simulink model "BMS_MIL_Wrapper"  (R2025b)
settings: Solver=ode3  StartTime=0.0  StopTime=20  FixedStep=.001  RelTol=1e-3  EnableMultiTasking=on
InitFcn:
  | battery_init;
  | Full_Charge_Volt=4.2; % unit volts
  | Cutoff_Volt=3; % unit volts
  | Delta=.02;
  | ContactorTime=20;
  | ContactorTimeOut=100;
  | High_TempLim=333;
  | Low_TempLim=263;
  | Sensor_Fault_Treshold=.02;
  | CurrentTimeout=1;
  | Allowed_Delta=.04;
  | Bal_On_Time=30;
  | Bal_Off_Time=5;
  | BalNotAct_Time=10;
values from neighbouring files (symbols this model uses):
  bonka_R0 = [ ... (first row only)    [battery_init.m]
  bonka_SOC = [0, 0.1, 0.2, 0.3, 0.4, 0.5, 0.6, 0.7, 0.8, 0.9, 1.0]    [battery_init.m]
  bonka_T = [263.15, 273.15, 298.15, 313.15, 328.15]    [battery_init.m]
  Charge_Rate = 1    [battery_init.m]
  Discharge_Rate = -1    [battery_init.m]
  Fly_Cycle_Current = [ ... (first row only)    [battery_init.m]
undefined symbols (not defined in the file or in its folder): DiscIntNeverNeededParam, From_Plant_MATLABStruct, SRE
libraries: fl_lib x69, nesl_utility x54, simulink x35, ee_lib x12, batteryecm_lib x12, BatteryCurrentManagement x1
(part 4 of 4)

== stateflow chart BMS_MIL_Wrapper/Test Sequence ==
  state Charging
    State_Required=SRE.Charge
  (default) -> Charging
  data: State_Required output Enum: SRE

== stateflow chart BMS_MIL_Wrapper/BMS_Closedloop/BMS_Control/Fault_Severity/Chart ==
  state UV_Fault_Severity
    during:
    if UV_Critical
    Fault_Level.UV = 4;
    elseif UV_Emergency
    Fault_Level.UV = 3;
    elseif UV_PowerLimit
    Fault_Level.UV = 2;
    elseif UV_Warning
    Fault_Level.UV = 1;
    else
    Fault_Level.UV = 0;
    end
  (default) -> UV_Fault_Severity
  data: UV_Warning input boolean; UV_PowerLimit input boolean; UV_Emergency input boolean; UV_Critical input boolean; Fault_Level output Bus: Fault_Level

== stateflow chart BMS_MIL_Wrapper/BMS_Closedloop/BMS_Control/Fault_Severity/Chart1 ==
  state UV_Fault_Severity
    during:
    if OV_Critical
    Fault_Level.OV = 3;
    elseif OV_Stop_Charge
    Fault_Level.OV = 2;
    elseif OV_Warning
    Fault_Level.OV= 1;
    else
    Fault_Level.OV = 0;
    end
  (default) -> UV_Fault_Severity
  data: OV_Warning input boolean; OV_Stop_Charge input boolean; OV_Critical input boolean; Fault_Level output Bus: Fault_Level

== stateflow chart BMS_MIL_Wrapper/BMS_Closedloop/BMS_Control/Fault_Severity/Chart2 ==
  state UV_Fault_Severity
    during:
    if OT_Critical
    Fault_Level.OT = 4;
    elseif OT_Emergency
    Fault_Level.OT = 3;
    elseif OT_PowerLimit
    Fault_Level.OT = 2;
    elseif OT_Warning
    Fault_Level.OT = 1;
    else
    Fault_Level.OT = 0;
    end
  (default) -> UV_Fault_Severity
  data: OT_Warning input boolean; OT_PowerLimit input boolean; OT_Emergency input boolean; OT_Critical input boolean; Fault_Level output Bus: Fault_Level

== stateflow chart BMS_MIL_Wrapper/BMS_Closedloop/BMS_Control/Fault_Severity/Chart3 ==
  state UV_Fault_Severity
    during:
    if UT_Critical
    Fault_Level.UT = 4;
    elseif UT_Emergency
    Fault_Level.UT = 3;
    elseif UT_PowerLimit
    Fault_Level.UT = 2;
    elseif UT_Warning
    Fault_Level.UT = 1;
    else
    Fault_Level.UT = 0;
    end
  (default) -> UV_Fault_Severity
  data: UT_Warning input boolean; UT_PowerLimit input boolean; UT_Emergency input boolean; UT_Critical input boolean; Fault_Level output Bus: Fault_Level

== stateflow chart BMS_MIL_Wrapper/BMS_Closedloop/BMS_Control/Subsystem/BMS_States ==
  state Fault_Monitoring [parallel]
    settings: executionOrder=2
    state Monitor_CurrentLim [parallel]
      settings: executionOrder=1
      state No_CurrentLim_Fault
      state Wait
      state OC_Fault
        en:
        FaultPresent=true;
        Fault_out.OC=true;
      (default) -> No_CurrentLim_Fault : {FaultPresent=false;
          |  Fault_out.OC=false;}
      No_CurrentLim_Fault -> Wait : [(Pack_Current< Current_Limits.Discharge_Current_Limit) || ...
          | (Pack_Current> Current_Limits.Charge_Current_Limit)]
      Wait -> No_CurrentLim_Fault [order 2] : [(Pack_Current >= Current_Limits.Discharge_Current_Limit) && ...
          | (Pack_Current <= Current_Limits.Charge_Current_Limit)]
      Wait -> OC_Fault [order 1] : [after(CurrentTimeout, sec)]
    state Monitor_CellVolt [parallel]
      settings: executionOrder=2
      state No_OV_UV
        en,du:
        Delta=abs(V_Batt_Sum-V_Batt_Monitor);
      state OV_Fault
        en:
        FaultPresent=true;
        Fault_out.OV=true;
      state UV_Fault
        en:
        FaultPresent=true;
        Fault_out.UV=true;
      state Sensor_Fault
        en:
        FaultPresent=true;
        Fault_out.VoltSensor=true;
      (default) -> No_OV_UV : {FaultPresent=false;
          | Fault_out.VoltSensor=false;
          | Fault_out.UV=false;
          | Fault_out.OV=false;}
      No_OV_UV -> OV_Fault [order 3] : [Max_Voltage>=Full_Charge_Volt]
      No_OV_UV -> (junction 190) [order 2] : [Min_Voltage <= Cutoff_Volt]
      (junction 190) -> UV_Fault
      No_OV_UV -> Sensor_Fault [order 1] : [Delta>=single(Sensor_Fault_Treshold)]
    state Monitor_CellTemp [parallel]
      settings: executionOrder=3
      state OT_Fault
        en:
        FaultPresent=true;
        Fault_out.OT=true;
      state No_OT_UT
        en, du:
        MaxCellTemp=max(Tmod);
        MinCellTemp=min(Tmod);
      state UT_Fault
        en:
        FaultPresent=true;
        Fault_out.UT=true;
      No_OT_UT -> OT_Fault [order 2] : [MaxCellTemp>=High_TempLim]
      (default) -> No_OT_UT : {FaultPresent=false;
          | Fault_out.OT=false;
          | Fault_out.UT=false;}
      No_OT_UT -> UT_Fault [order 1] : [MinCellTemp<=Low_TempLim]
  state Normal_State [parallel]
    settings: executionOrder=1
    state Standby
      en:
      BMS_State_Out= BMS_State.Standbying
    state Charging
      en:
      BMS_State_Out= BMS_State.Charging
    state Flying
      en:
      BMS_State_Out= BMS_State.Flying
    state Fault
      en,du:
      BMS_State_Out= BMS_State.Fault
    (default) -> Standby
    Standby -> Charging [order 2] : [State_Required==SRE.Charge ]
    Standby -> (junction 206) [order 3] : [FaultPresent]
    (junction 206) -> (junction 209)
    Charging -> Standby [order 1] : [(State_Required~=SRE.Charge)...
        | || (State_Required==SRE.Standby) ]
    Standby -> Flying [order 1] : [State_Required== SRE.Fly]
    Flying -> Standby [order 1] : [(State_Required~=SRE.Fly) ||...
        | (State_Required==SRE.Standby) ]
    (junction 207) -> Charging
    Charging -> (junction 208) [order 2]
    Charging -> Fault [order 3] : [FaultPresent]
    Flying -> (junction 207) [order 2] : [State_Required==SRE.Charge]
    (junction 208) -> Flying : [State_Required== SRE.Fly]
    Flying -> Fault [order 3] : [FaultPresent]
    (junction 209) -> Fault
  data: Current_Limits input Bus: Current_Limits; Tmod input single; V_Batt_Sum input; Pack_Current input single; V_Batt_Monitor input; State_Required input Enum: SRE; Fault_out output Bus: Fault_out; Max_Voltage input single; Min_Voltage input single; Low_TempLim parameter single; High_TempLim parameter single; Cutoff_Volt parameter single; Full_Charge_Volt parameter single; MaxCellTemp local single; MinCellTemp local single; Delta local single; Sensor_Fault_Treshold parameter double; FaultPresent local boolean; BMS_State_Out output Enum: BMS_State; CurrentTimeout parameter

== stateflow chart BMS_MIL_Wrapper/BMS_Closedloop/BMS_Control/Subsystem1/Chart ==
  state Balancing_Off
    en:
    Bal_Cmd(:,:)= false;
    en, du:
    DeltaCellVolt=Max_Voltage-Min_Voltage;
  state Balancing_On
    en, du:
    DeltaCellVolt=Max_Voltage-Min_Voltage;
    state Balance_Active
      en, du:
      Bal_Cmd=((Vmod-Min_Voltage)> Allowed_Delta/2)';
      flgBalCompl=all(~Bal_Cmd);
    state Balance_Not_Active
    (default) -> Balance_Active
    Balance_Not_Active -> Balance_Active [order 1] : [after(BalNotAct_Time, sec) &&...
        |  DeltaCellVolt> Allowed_Delta]
    Balance_Active -> Balance_Not_Active : [flgBalCompl]
  (default) -> Balancing_Off : {flgBalCompl=true}
  Balancing_Off -> Balancing_On : [flgBalInt &&...
      | BMS_State_Out==BMS_State.Charging &&...
      | after(Bal_Off_Time, sec) &&...
      | DeltaCellVolt> Allowed_Delta]
  Balancing_On -> Balancing_Off : [BMS_State_Out==BMS_State.Flying]
  Balance_Not_Active -> Balancing_Off [order 2] : [after(Bal_On_Time, sec)]
  data: BMS_State_Out input; Min_Voltage input single; Max_Voltage input single; Bal_Cmd output boolean; Allowed_Delta parameter single; DeltaCellVolt local single; Bal_On_Time parameter single; Bal_Off_Time parameter single; BalNotAct_Time parameter single; Vmod input single; flgBalCompl local boolean =false; flgBalInt local =true

== stateflow chart BMS_MIL_Wrapper/BMS_Closedloop/FC/Chart ==
  state Needed_Action
    if Fault_Level == 4
    Drone_Mode = 4;
    Motor_Command = 0;
    elseif Fault_Level == 3
    Drone_Mode = 3;
    Motor_Command = 0.3;
    elseif Fault_Level == 2
    Drone_Mode = 2;
    Motor_Command = 0.6;
    elseif Fault_Level == 1
    Drone_Mode = 1;
    Motor_Command = 1.0;
    else
    Drone_Mode = 0;
    Motor_Command = 1.0;
    end
  (default) -> Needed_Action
  data: Drone_Mode output; Motor_Command output; Fault_Level input
